simulink model "s61"  (R2016a)
settings: Solver=VariableStepAuto  StartTime=0.0  StopTime=10.0  RelTol=1e-3
settings Model: Creator=asifa  LastModifiedBy=asifa

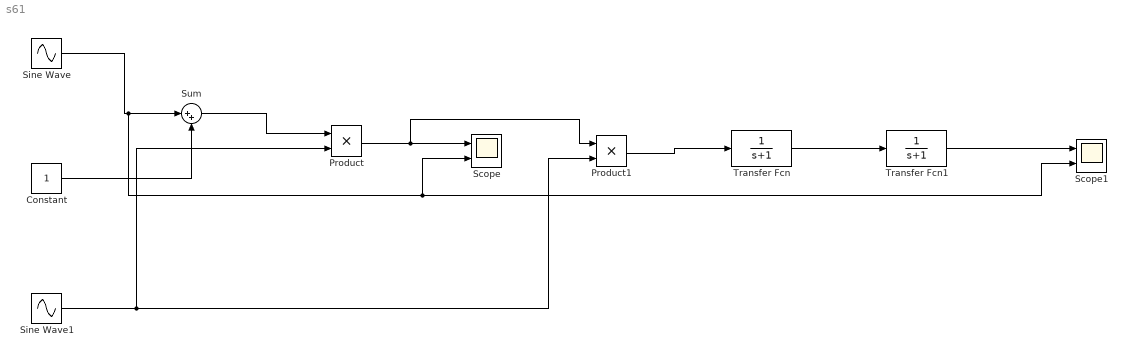
== system s61 ==
  Constant : Constant
  Product : Product
  Product1 : Product
  Scope : Scope  NumInputPorts=2
  Scope1 : Scope  NumInputPorts=2
  Sine Wave : Sin  Frequency=2*pi*25  SampleTime=1/5000
  Sine Wave1 : Sin  Frequency=2*pi  SampleTime=1/5000
  Sum : Sum  Inputs=|++
  Transfer Fcn : TransferFcn  Denominator=[1 1]
  Transfer Fcn1 : TransferFcn  Denominator=[1 1]
  wires:
  Sine Wave/1 -> Scope1/2, Scope/2, Sum/1
  Constant/1 -> Sum/2
  Sum/1 -> Product/1
  Sine Wave1/1 -> Product/2, Product1/2
  Product/1 -> Scope/1, Product1/1
  Product1/1 -> Transfer Fcn/1
  Transfer Fcn/1 -> Transfer Fcn1/1
  Transfer Fcn1/1 -> Scope1/1
